simulink model "sender_task"  (Simulink 3.00)
libraries: genlib x2, mathlib x2, speclib x1

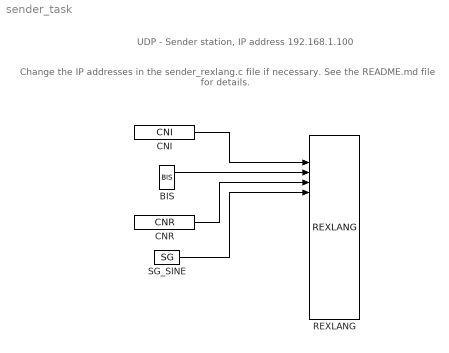
== system sender_task ==
  note: Change the IP addresses in the sender_rexlang.c file if necessary.
      |
      | See the README.md file for details.
  note: UDP - Sender station, IP address 192.168.1.100
  BIS : genlib/BIS  Y0=off  t1=1  t2=2  t3=0  t4=4  t5=5  t6=6  t7=7  t8=8  RPT=on
  CNI : mathlib/CNI  icn=87654321
  CNR : mathlib/CNR  ycn=-247.18
  REXLANG : speclib/REXLANG  srcname=sender_rexlang.c  srctype=1: C-like  debug=3: Full check  stack=0  strs=0
  SG_SINE : genlib/SG  isig=1: SINE  amp=10  freq=0.03  phase=0  ifrunit=1: Hz  iphunit=1: degrees  offset=0
  wires:
  BIS/1 -> REXLANG/4
  CNI/1 -> REXLANG/3
  CNR/1 -> REXLANG/5
  SG_SINE/1 -> REXLANG/6
